simulink model "EulerAnglesFromAngularVelocity"  (R2016a)
settings: Solver=VariableStepAuto  SolverMode=SingleTasking  StartTime=0.0  StopTime=10.0  RelTol=1e-3
undefined symbols (not defined in the file): DiscIntNeverNeededParam
settings Model: Creator=Alireza  LastModifiedBy=Alireza
settings DataIOCC: ReturnWorkspaceOutputs=on
settings DebuggingCC: SFUnexpectedBacktrackingDiag=error  SFNoUnconditionalDefaultTransitionDiag=error
settings SFSimCC: SimUseLocalCustomCode=on
settings RTWCC: RTWUseLocalCustomCode=on
settings GRTTargetCC: TargetLangStandard=C99 (ISO)
settings ConfigComp: CovMetricSettings=dwe  CovHtmlReporting=off  CovSaveCumulativeToWorkspaceVar=off  CovSaveSingleToWorkspaceVar=off  CovExternalEMLEnable=on

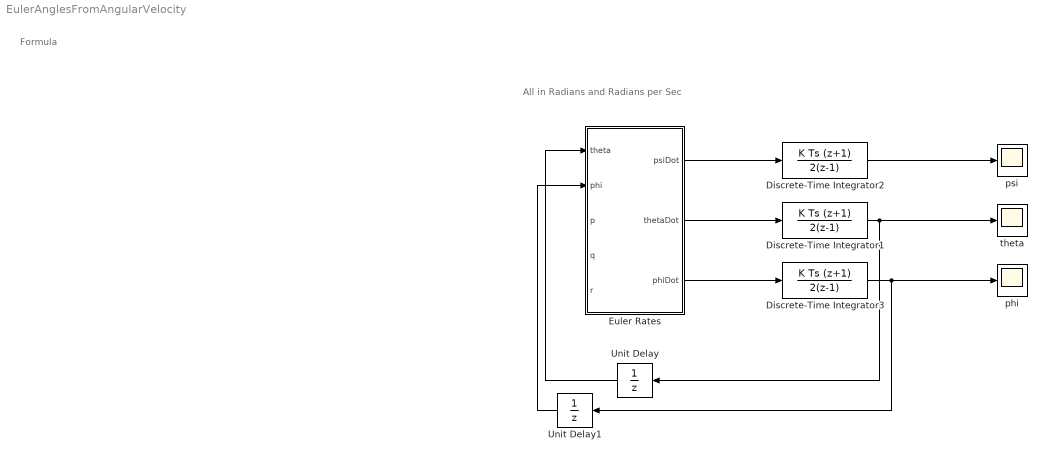
== system EulerAnglesFromAngularVelocity ==
  note: Formula
  note: All in Radians and Radians per Sec
  Discrete-Time Integrator1 : DiscreteIntegrator  IntegratorMethod=Integration: Trapezoidal  InitialConditionSetting=State (most efficient)  SampleTime=-1  ICPrevOutput=DiscIntNeverNeededParam  ICPrevScaledInput=DiscIntNeverNeededParam
  Discrete-Time Integrator2 : DiscreteIntegrator  IntegratorMethod=Integration: Trapezoidal  InitialConditionSetting=State (most efficient)  SampleTime=-1  ICPrevOutput=DiscIntNeverNeededParam  ICPrevScaledInput=DiscIntNeverNeededParam
  Discrete-Time Integrator3 : DiscreteIntegrator  IntegratorMethod=Integration: Trapezoidal  InitialConditionSetting=State (most efficient)  SampleTime=-1  ICPrevOutput=DiscIntNeverNeededParam  ICPrevScaledInput=DiscIntNeverNeededParam
  Euler Rates : Subsystem
  Unit Delay : UnitDelay  SampleTime=-1  HasFrameUpgradeWarning=on
  Unit Delay1 : UnitDelay  SampleTime=-1  HasFrameUpgradeWarning=on
  phi : Scope
  psi : Scope
  theta : Scope
  wires:
  Euler Rates/2(thetaDot) -> Discrete-Time Integrator1/1
  Unit Delay1/1 -> Euler Rates/2(phi)
  Unit Delay/1 -> Euler Rates/1(theta)
  Euler Rates/3(phiDot) -> Discrete-Time Integrator3/1
  Euler Rates/1(psiDot) -> Discrete-Time Integrator2/1
  Discrete-Time Integrator3/1 -> Unit Delay1/1, phi/1
  Discrete-Time Integrator1/1 -> theta/1, Unit Delay/1
  Discrete-Time Integrator2/1 -> psi/1

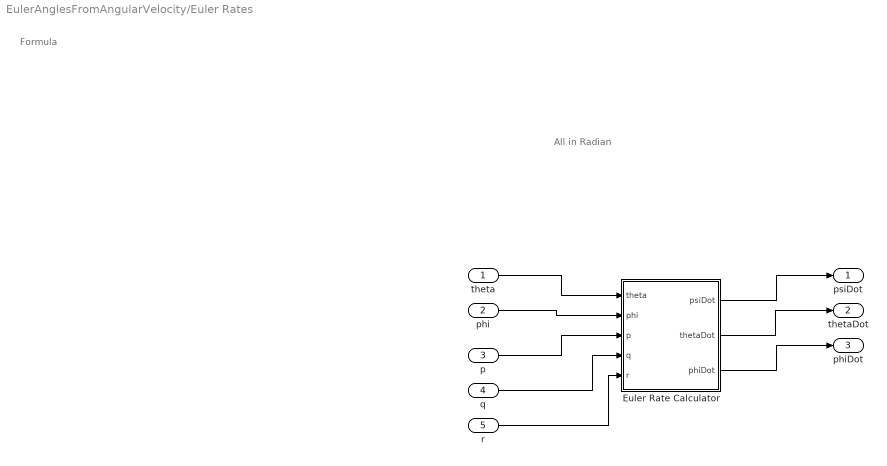
== system EulerAnglesFromAngularVelocity/Euler Rates ==
  note: All in Radian
  note: Formula
  theta : Inport
  phi : Inport  Port=2
  p : Inport  Port=3
  q : Inport  Port=4
  r : Inport  Port=5
  Euler Rate Calculator : MATLAB Function  TreatAsAtomicUnit=on
  psiDot : Outport
  thetaDot : Outport  Port=2
  phiDot : Outport  Port=3
  wires:
  phi/1 -> Euler Rate Calculator/2(phi)
  theta/1 -> Euler Rate Calculator/1(theta)
  p/1 -> Euler Rate Calculator/3(p)
  q/1 -> Euler Rate Calculator/4(q)
  r/1 -> Euler Rate Calculator/5(r)
  Euler Rate Calculator/1(psiDot) -> psiDot/1
  Euler Rate Calculator/2(thetaDot) -> thetaDot/1
  Euler Rate Calculator/3(phiDot) -> phiDot/1

== matlab function EulerAnglesFromAngularVelocity/Euler Rates/Euler Rate Calculator ==
  data: theta input; psiDot output; phi input; p input; q input; r input; thetaDot output; phiDot output
function [psiDot,thetaDot,phiDot] = fcn(theta,phi,p,q,r)

psiDot =  sin(phi)/cos(theta)*q + cos(phi)/cos(theta)*r;
thetaDot = cos(phi)*q - sin(phi)*r;
phiDot = p + sin(phi)*tan(theta)*q + cos(phi)*tan(theta)*r;
end
